simulink model "testTemperatureSwitch"  (R2016b)
settings: Solver=FixedStepAuto  StartTime=0.0  StopTime=100  FixedStep=0.002  RelTol=1e-3
libraries: TemperatureSwitch x1
settings Model: Creator=Marc  LastModifiedBy=Marc

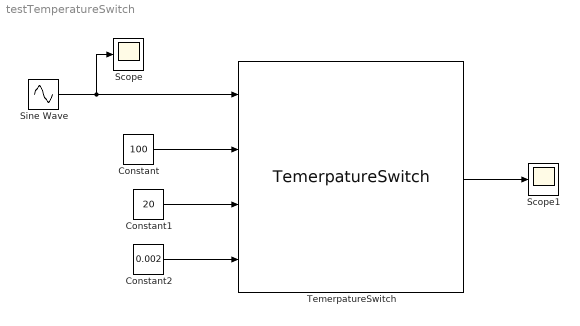
== system testTemperatureSwitch ==
  Constant : Constant  Value=100
  Constant1 : Constant  Value=20
  Constant2 : Constant  Value=0.002
  Scope : Scope
  Scope1 : Scope
  Sine Wave : Sin  Amplitude=1000  Frequency=0.01  SampleTime=0.002
  TemerpatureSwitch : TemperatureSwitch/TemerpatureSwitch
  wires:
  Constant1/1 -> TemerpatureSwitch/3
  Constant/1 -> TemerpatureSwitch/2
  Constant2/1 -> TemerpatureSwitch/4
  Sine Wave/1 -> TemerpatureSwitch/1, Scope/1
  TemerpatureSwitch/1 -> Scope1/1
